simulink model "example_block"  (R2022b)
settings: Solver=VariableStepAuto  StartTime=0.0  StopTime=10.0  RelTol=1e-3
values from neighbouring files (symbols this model uses):
  b = 1.523    [example.m]
  k1 = 1    [example.m]
  k2 = 19.8    [example.m]
  m = 0.65    [example.m]    (also in state_vector_feedback_example.m = 0.5)
settings Model: Creator=cotti  LastModifiedBy=cotti

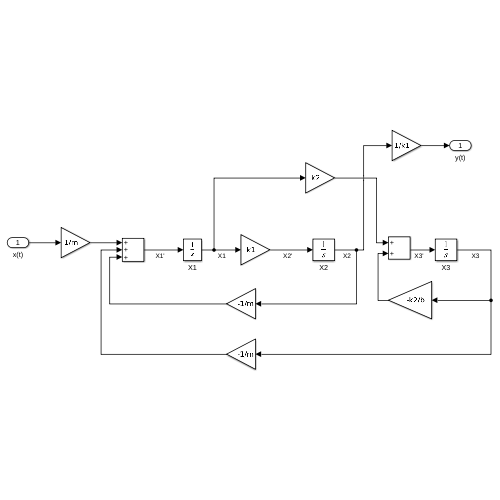
[thumbnail: Simulink's stored preview of the top-level diagram]
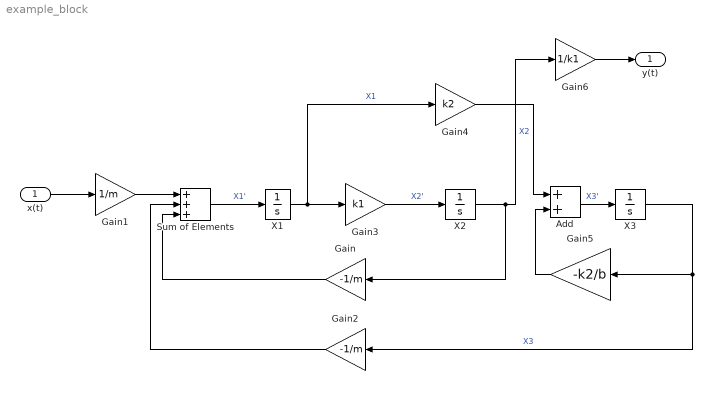
== system example_block ==
  x(t) : Inport
  Add : Sum
  Gain : Gain  Gain=-1/m
  Gain1 : Gain  Gain=1/m
  Gain2 : Gain  Gain=-1/m
  Gain3 : Gain  Gain=k1
  Gain4 : Gain  Gain=k2
  Gain5 : Gain  Gain=-k2/b
  Gain6 : Gain  Gain=1/k1
  Sum of Elements : Sum  Inputs=+++
  X1 : Integrator
  X2 : Integrator
  X3 : Integrator
  y(t) : Outport
  wires:
  X1/1 -> Gain4/1, Gain3/1  "X1"
  Gain3/1 -> X2/1  "X2'"
  X2/1 -> Gain6/1, Gain/1  "X2"
  Sum of Elements/1 -> X1/1  "X1'"
  Gain/1 -> Sum of Elements/3
  x(t)/1 -> Gain1/1
  Gain1/1 -> Sum of Elements/1
  X3/1 -> Gain5/1, Gain2/1  "X3"
  Gain2/1 -> Sum of Elements/2
  Gain5/1 -> Add/2
  Gain4/1 -> Add/1
  Gain6/1 -> y(t)/1
  Add/1 -> X3/1  "X3'"
